simulink model "IBC_DCM_Test"  (R2019b)
settings: Solver=VariableStepAuto  StartTime=0.0  StopTime=0.03  RelTol=1e-3
InitFcn:
  | Load=2;
  | C=370e-6;
  | L1=1000e-6;
  | L2=1000e-6*(1+normrnd(0,0.05,[1,1]));
  | L3=1000e-6*(1+normrnd(0,0.05,[1,1]));
  | alp=1-0.5;
  | V = 12;
  | L = 1000e-6;
  | D = 0.5;
  | Vg= 12;
  | R = 2;
libraries: powerlib x23, simulink x12, dspsigops x5, powerlib_meascontrol x2
settings Model: SimulationMode=accelerator  Creator=29721  LastModifiedBy=29721

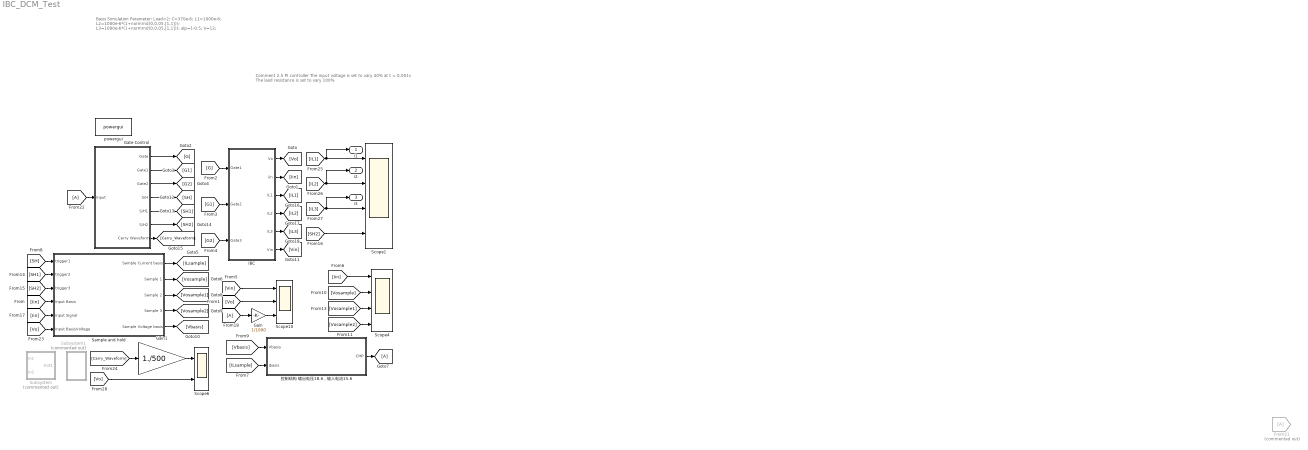
== system IBC_DCM_Test ==
  note: Comment 2.5
      | PI controller
      | The input voltage is set to vary 40% at t = 0.001s
      | The laod resistance is set to vary 100%
  note: Basis Simulation
      | Parameter:
      | Load=2;
      | C=370e-6;
      | L1=1000e-6;
      | L2=1000e-6*(1+normrnd(0,0.05,[1,1]));
      | L3=1000e-6*(1+normrnd(0,0.05,[1,1]));
      | alp=1-0.5;
      | V=12;
  From21 : From  Commented=on
  Gain : Gain  Gain=1/1000
  Gain1 : Gain  Gain=1./500
  Gate Control : Subsystem  mask{Fs=10e3}
      mask prompts: Fs "swicthing frequency"
  IBC : Subsystem  mask{L1=L1, L2=L1, L3=L1, C=C, R=R, Vin=Vg}
  "Sample and hold " : Subsystem
  Scope1 : Scope  NumInputPorts=4
  Scope10 : Scope  NumInputPorts=3
  Scope4 : Scope  NumInputPorts=4
  Scope6 : Scope  NumInputPorts=2
  Subsystem : Subsystem  Commented=on
  Subsystem1 : Subsystem  Commented=on
  powergui : powerlib/powergui  Priority=1  SimulationMode=Discrete  SampleTime=2.5e-8  frequency=60  Iterations=50  frequencyindice=0  Pbase=100e6  ErrMax=1e-4  UnitsV=kV  UnitsW=MW  buscounter=0  FunctionMessages=off  echomessages=off  EnableUseOfTLC=off  CurrentSourceSwitches=off  DisableSnubberDevices=off  DisableRonSwitches=off  DisableVfSwitches=off  DisplayEquations=off  AutomaticDiscreteSolvers=off  SolverType=Tustin/Backward Euler (TBE)  Interpol=off  ExternalGateDelay=off  methode=off  Ts=100  x0status=blocks  SPID=on  SwTol=0  HookPort=off  NonlinearTolerance=1e-4  nMaxIteration=100  ContinueOnMaxIteration=off  RestoreLinks=warning  ResistiveCurrentMeasurement=off  Frange=[0:2:500]  Ylog=off  Xlog=on  ShowGrid=off  save=off  variable=ZData  structure=0  ZoomFFT=off  StartTime=0.0  cycles=1  DisplayStyle=1  fundamental=60  FreqAxis=off  MaxFrequency=1000  frequencyindicesteady=1  RmsSteady=1  display=off
      settings: SourceProductName=Simscape Electrical
  控制结构 输出电压18.6，输入电流15.6 : Subsystem
  i1 : Outport
  i2 : Outport  Port=2
  i3 : Outport  Port=3
  wires:
  [Vosample1] -> Scope4/3
  [Vosample2] -> Scope4/4
  [Vin] -> Scope10/1
  [Vo] -> Scope10/2
  [Vosample] -> Scope4/2
  Gain1/1 -> Scope6/1
  [SH2] -> "Sample and hold "/3(trigger3)
  [Carry_Waveform] -> Gain1/1
  Gate Control/1(Gate) -> [G]
  Gate Control/2(Gate1) -> [G1]
  Gate Control/3(Gate2) -> [G2]
  [SH] -> "Sample and hold "/1(trigger1)
  [SH1] -> "Sample and hold "/2(trigger2)
  [Iin] -> "Sample and hold "/4(Input Basis)
  "Sample and hold "/1(Sample Current basis) -> [ILsample]
  "Sample and hold "/2(Sample 1) -> [Vosample]
  "Sample and hold "/3(Sample 2) -> [Vosample1]
  "Sample and hold "/4(Sample 3) -> [Vosample2]
  [Iin] -> Scope4/1
  [A] -> Gain/1
  "Sample and hold "/5(Sample Voltage basis) -> [Vbasis]
  [IL1] -> i1/1, Scope1/1
  [IL2] -> i2/1, Scope1/2
  [IL3] -> i3/1, Scope1/3
  [G] -> IBC/1(Gate1)
  [G1] -> IBC/2(Gate2)
  [G2] -> IBC/3(Gate3)
  IBC/1(Vo) -> [Vo]
  IBC/2(Iin) -> [Iin]
  [A] -> Gate Control/1(Input)
  Gate Control/4(S/H) -> [SH]
  Gate Control/5(S/H1) -> [SH1]
  Gate Control/6(S/H2) -> [SH2]
  [SH2] -> Scope1/4
  [Iin] -> "Sample and hold "/5(Input Signal)
  [Vo] -> "Sample and hold "/6(Input BasisVoltage)
  Gate Control/7(Carry Waveform) -> [Carry_Waveform]
  IBC/3(IL1) -> [IL1]
  IBC/4(IL2) -> [IL2]
  IBC/5(IL3) -> [IL3]
  [Vo] -> Scope6/2
  控制结构 输出电压18.6，输入电流15.6/1("CMP ") -> [A]
  [Vbasis] -> 控制结构 输出电压18.6，输入电流15.6/1(Vbasis)
  [ILsample] -> 控制结构 输出电压18.6，输入电流15.6/2(Ibasis)
  Gain/1 -> Scope10/3
  IBC/6(Vin) -> [Vin]

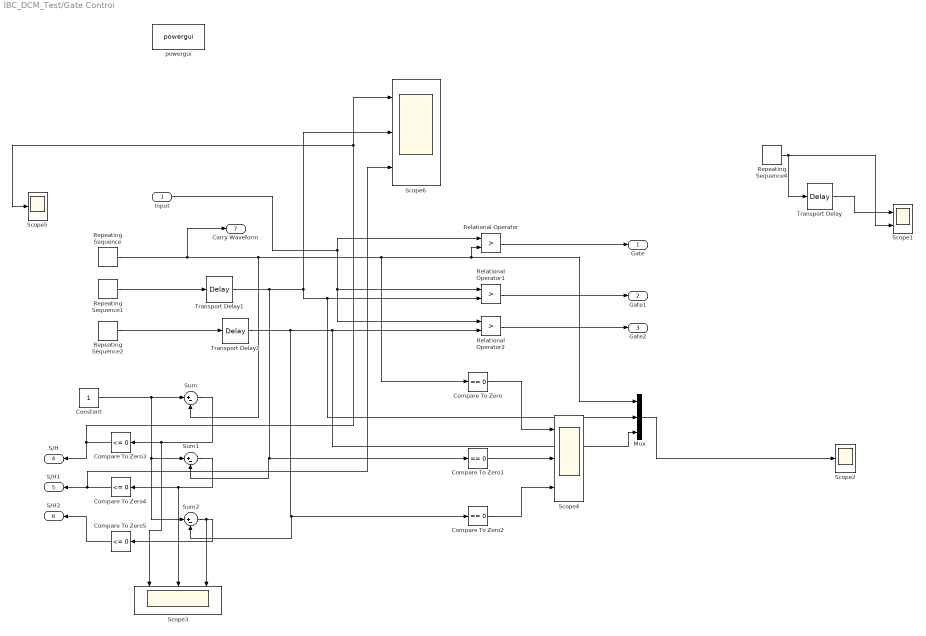
== system IBC_DCM_Test/Gate Control ==
  Input : Inport
  Compare To Zero : simulink/Logic and Bit Operations/Compare To Zero  relop===  OutDataTypeStr=boolean
  Compare To Zero1 : simulink/Logic and Bit Operations/Compare To Zero  relop===  OutDataTypeStr=boolean
  Compare To Zero2 : simulink/Logic and Bit Operations/Compare To Zero  relop===  OutDataTypeStr=boolean
  Compare To Zero3 : simulink/Logic and Bit Operations/Compare To Zero  relop=<=  OutDataTypeStr=boolean
  Compare To Zero4 : simulink/Logic and Bit Operations/Compare To Zero  relop=<=  OutDataTypeStr=boolean
  Compare To Zero5 : simulink/Logic and Bit Operations/Compare To Zero  relop=<=  OutDataTypeStr=boolean
  Constant : Constant
  Mux : Mux  Inputs=3
  Relational Operator : RelationalOperator  Operator=>  OutDataTypeStr=boolean  RndMeth=Simplest
  Relational Operator1 : RelationalOperator  Operator=>  OutDataTypeStr=boolean  RndMeth=Simplest
  Relational Operator2 : RelationalOperator  Operator=>  OutDataTypeStr=boolean  RndMeth=Simplest
  Repeating Sequence : simulink/Sources/Repeating Sequence  rep_seq_t=[0 1./Fs./2 1./Fs]  rep_seq_y=[0 1000 0]
  Repeating Sequence1 : simulink/Sources/Repeating Sequence  rep_seq_t=[1./Fs./3 5./Fs./6 4./Fs./3]  rep_seq_y=[0 1000 0]
  Repeating Sequence2 : simulink/Sources/Repeating Sequence  rep_seq_t=[2./Fs./3 7./Fs./6 5./Fs./3]  rep_seq_y=[0 1000 0]
  Repeating Sequence4 : simulink/Sources/Repeating Sequence  rep_seq_t=[0 1./100e3./2 1./100e3]  rep_seq_y=[0 1000 0]
  Scope1 : Scope  NumInputPorts=2
  Scope2 : Scope
  Scope3 : Scope  NumInputPorts=3
  Scope4 : Scope  NumInputPorts=3
  Scope5 : Scope
  Scope6 : Scope  NumInputPorts=3
  Sum : Sum  Inputs=|+-
  Sum1 : Sum  Inputs=|+-
  Sum2 : Sum  Inputs=|+-
  Transport Delay : TransportDelay  DelayTime=1./100e3./3
  Transport Delay1 : TransportDelay  DelayTime=1./Fs./3
  Transport Delay2 : TransportDelay  DelayTime=2./Fs./3
  powergui : powerlib/powergui  Priority=1  SimulationMode=Discrete  SampleTime=2.5e-8  frequency=60  Iterations=50  frequencyindice=60  Pbase=100e6  ErrMax=1e-4  UnitsV=kV  UnitsW=MW  buscounter=0  FunctionMessages=off  echomessages=off  EnableUseOfTLC=off  CurrentSourceSwitches=off  DisableSnubberDevices=off  DisableRonSwitches=off  DisableVfSwitches=off  DisplayEquations=off  AutomaticDiscreteSolvers=off  SolverType=Tustin/Backward Euler (TBE)  Interpol=off  ExternalGateDelay=off  methode=off  Ts=100  x0status=blocks  SPID=on  SwTol=0  HookPort=off  NonlinearTolerance=1e-4  nMaxIteration=100  ContinueOnMaxIteration=off  RestoreLinks=warning  ResistiveCurrentMeasurement=off  Frange=[0:2:500]  Ylog=off  Xlog=on  ShowGrid=off  save=off  variable=ZData  structure=0  ZoomFFT=off  StartTime=0.0  cycles=1  DisplayStyle=1  fundamental=60  FreqAxis=off  MaxFrequency=1000  frequencyindicesteady=1  RmsSteady=1  display=off
      settings: SourceProductName=Simscape Electrical
  Gate : Outport
  Gate1 : Outport  Port=2
  Gate2 : Outport  Port=3
  S/H : Outport  Port=4
  S/H1 : Outport  Port=5
  S/H2 : Outport  Port=6
  Carry Waveform : Outport  Port=7
  wires:
  Input/1 -> Relational Operator1/1, Relational Operator2/1, Relational Operator/1
  Compare To Zero/1 -> Scope4/1
  Relational Operator/1 -> Gate/1
  Repeating Sequence1/1 -> Transport Delay1/1
  Relational Operator1/1 -> Gate1/1
  Repeating Sequence2/1 -> Transport Delay2/1
  Repeating Sequence/1 -> Carry Waveform/1, Mux/1, Relational Operator/2, Compare To Zero/1, Sum/2
  Relational Operator2/1 -> Gate2/1
  Repeating Sequence4/1 -> Transport Delay/1, Scope1/2
  Transport Delay/1 -> Scope1/1
  Mux/1 -> Scope2/1
  Transport Delay1/1 -> Sum1/2, Compare To Zero1/1, Scope6/2, Mux/2, Relational Operator1/2
  Compare To Zero1/1 -> Scope4/2
  Compare To Zero2/1 -> Scope4/3
  Sum/1 -> Scope3/1, Compare To Zero3/1
  Sum1/1 -> Compare To Zero4/1, Scope3/2
  Transport Delay2/1 -> Sum2/2, Compare To Zero2/1, Mux/3, Relational Operator2/2
  Sum2/1 -> Scope3/3, Compare To Zero5/1
  Constant/1 -> Sum2/1, Sum1/1, Sum/1
  Compare To Zero3/1 -> Scope6/1, Scope5/1, S/H/1
  Compare To Zero4/1 -> Scope6/3, S/H1/1
  Compare To Zero5/1 -> S/H2/1

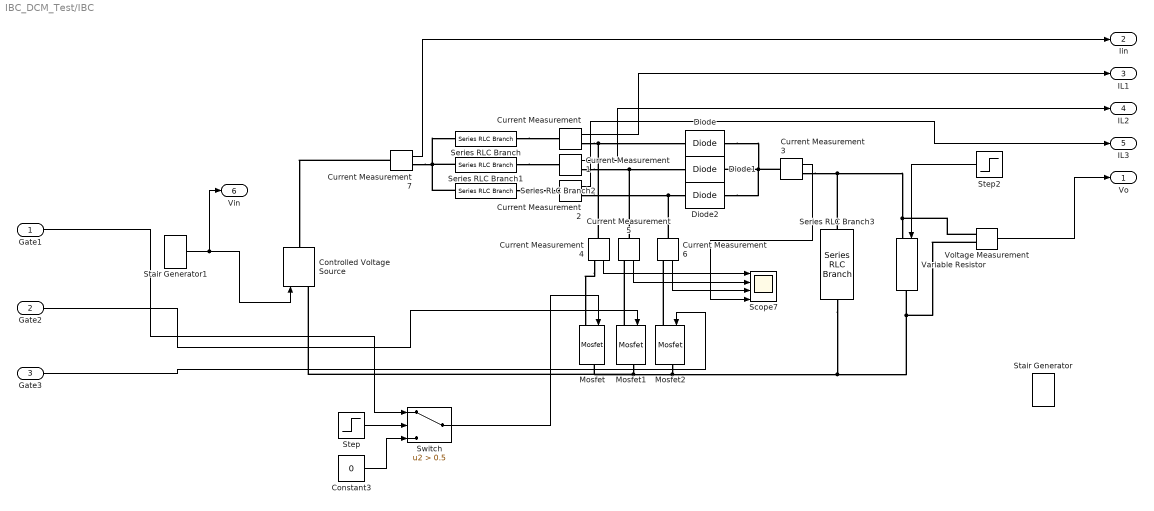
== system IBC_DCM_Test/IBC ==
  Gate1 : Inport
  Gate2 : Inport  Port=2
  Gate3 : Inport  Port=3
  Constant3 : Constant  Value=0
  Controlled Voltage Source : powerlib/Electrical Sources/Controlled Voltage Source  Initialize=on  Source_Type=AC  Amplitude=0  Phase=0  Frequency=0  Measurements=None
      settings: SourceProductName=Simscape Electrical
  Current Measurement{,1..7} (8 alike) : powerlib/Measurements/Current Measurement  PhasorSimulation=off  OutputType=Complex  PSBequivalent=0
      settings: SourceProductName=Simscape Electrical
  Diode : powerlib/Power Electronics/Diode  Ron=0.001  Lon=0  Vf=0  IC=0  UseSnubber=0  Rs=inf  Cs=250e-9  Measurements=off
      settings: SourceProductName=Simscape Electrical
  Diode1 : powerlib/Power Electronics/Diode  Ron=0.001  Lon=0  Vf=0  IC=0  UseSnubber=0  Rs=inf  Cs=250e-9  Measurements=off
      settings: SourceProductName=Simscape Electrical
  Diode2 : powerlib/Power Electronics/Diode  Ron=0.001  Lon=0  Vf=0  IC=0  UseSnubber=0  Rs=inf  Cs=250e-9  Measurements=off
      settings: SourceProductName=Simscape Electrical
  Mosfet : powerlib/Power Electronics/Mosfet  Ron=0.01  Lon=0  Rd=0.01  Vfd=0  IC=0  Rs=1e5  Cs=inf  Measurements=off
      settings: SourceProductName=Simscape Electrical
  Mosfet1 : powerlib/Power Electronics/Mosfet  Ron=0.01  Lon=0  Rd=0.01  Vfd=0  IC=0  Rs=1e5  Cs=inf  Measurements=off
      settings: SourceProductName=Simscape Electrical
  Mosfet2 : powerlib/Power Electronics/Mosfet  Ron=0.01  Lon=0  Rd=0.01  Vfd=0  IC=0  Rs=1e5  Cs=inf  Measurements=off
      settings: SourceProductName=Simscape Electrical
  Scope7 : Scope  NumInputPorts=4
  Series RLC Branch : powerlib/Elements/Series RLC Branch  LConnTagsString=__new0  RConnTagsString=__new0  BranchType=L  Resistance=1  Inductance=L1  SetiL0=off  InitialCurrent=0  Capacitance=1e-6  Setx0=off  InitialVoltage=0  Measurements=None
      settings: SourceProductName=Simscape Electrical
  Series RLC Branch1 : powerlib/Elements/Series RLC Branch  LConnTagsString=__new0  RConnTagsString=__new0  BranchType=L  Resistance=1  Inductance=L2  SetiL0=off  InitialCurrent=0  Capacitance=1e-6  Setx0=off  InitialVoltage=0  Measurements=None
      settings: SourceProductName=Simscape Electrical
  Series RLC Branch2 : powerlib/Elements/Series RLC Branch  LConnTagsString=__new0  RConnTagsString=__new0  BranchType=L  Resistance=1  Inductance=L3  SetiL0=off  InitialCurrent=0  Capacitance=1e-6  Setx0=off  InitialVoltage=0  Measurements=None
      settings: SourceProductName=Simscape Electrical
  Series RLC Branch3 : powerlib/Elements/Series RLC Branch  LConnTagsString=__new0  RConnTagsString=__new0  BranchType=RC  Resistance=0  Inductance=1e-3  SetiL0=off  InitialCurrent=0  Capacitance=C  Setx0=off  InitialVoltage=0  Measurements=None
      settings: SourceProductName=Simscape Electrical
  Stair Generator : powerlib_meascontrol/Pulse & Signal Generators/Stair Generator  t=[0,0.01,0.02]  e=[2,4,8]  Ts=0
      settings: SourceProductName=Simscape Electrical
  Stair Generator1 : powerlib_meascontrol/Pulse & Signal Generators/Stair Generator  t=[0,0.01,0.02]  e=[10,10,10]  Ts=0
      settings: SourceProductName=Simscape Electrical
  Step : Step  Time=0.025  Before=1  After=0  SampleTime=0
  Step2 : Step  Time=0.01  Before=4  After=6  SampleTime=0
  Switch : Switch  Criteria=u2 > Threshold  Threshold=0.5
  Variable Resistor : powerlib/Elements/Variable Resistor  Rabsmin=1e-3
      settings: SourceProductName=Simscape Electrical  SourceProductBaseCode=PS
  Voltage Measurement : powerlib/Measurements/Voltage Measurement  PhasorSimulation=off  OutputType=Complex  PSBequivalent=0
      settings: SourceProductName=Simscape Electrical
  Vo : Outport
  Iin : Outport  Port=2
  IL1 : Outport  Port=3
  IL2 : Outport  Port=4
  IL3 : Outport  Port=5
  Vin : Outport  Port=6
  wires:
  Step2/1 -> Variable Resistor/1
  Current Measurement6/1 -> Scope7/3
  Current Measurement5/1 -> Scope7/2
  Current Measurement1/1 -> IL2/1
  Current Measurement4/1 -> Scope7/1
  Current Measurement2/1 -> IL3/1
  Step/1 -> Switch/2
  Switch/1 -> Mosfet/1
  Current Measurement3/1 -> Scope7/4
  Stair Generator1/1 -> Vin/1, Controlled Voltage Source/1
  Gate3/1 -> Mosfet2/1
  Voltage Measurement/1 -> Vo/1
  Current Measurement/1 -> IL1/1
  Constant3/1 -> Switch/3
  Current Measurement7/1 -> Iin/1
  Gate1/1 -> Switch/1
  Gate2/1 -> Mosfet1/1
  connections:
  Series RLC Branch2/RConn1 -- Current Measurement2/LConn1
  Mosfet2/LConn1 -- Current Measurement6/RConn1
  Current Measurement7/LConn1 -- Controlled Voltage Source/RConn1
  Series RLC Branch/RConn1 -- Current Measurement/LConn1
  Series RLC Branch1/RConn1 -- Current Measurement1/LConn1
  Controlled Voltage Source/LConn1 -- Mosfet/RConn1 -- Mosfet1/RConn1 -- Mosfet2/RConn1 -- Voltage Measurement/LConn2 -- Variable Resistor/RConn1 -- Series RLC Branch3/RConn1
  Mosfet1/LConn1 -- Current Measurement5/RConn1
  Current Measurement2/RConn1 -- Current Measurement6/LConn1 -- Diode2/LConn1
  Current Measurement3/RConn1 -- Series RLC Branch3/LConn1 -- Voltage Measurement/LConn1 -- Variable Resistor/LConn1
  Current Measurement4/RConn1 -- Mosfet/LConn1
  Current Measurement7/RConn1 -- Series RLC Branch2/LConn1 -- Series RLC Branch1/LConn1 -- Series RLC Branch/LConn1
  Current Measurement1/RConn1 -- Diode1/LConn1 -- Current Measurement5/LConn1
  Current Measurement3/LConn1 -- Diode2/RConn1 -- Diode/RConn1 -- Diode1/RConn1
  Current Measurement/RConn1 -- Diode/LConn1 -- Current Measurement4/LConn1

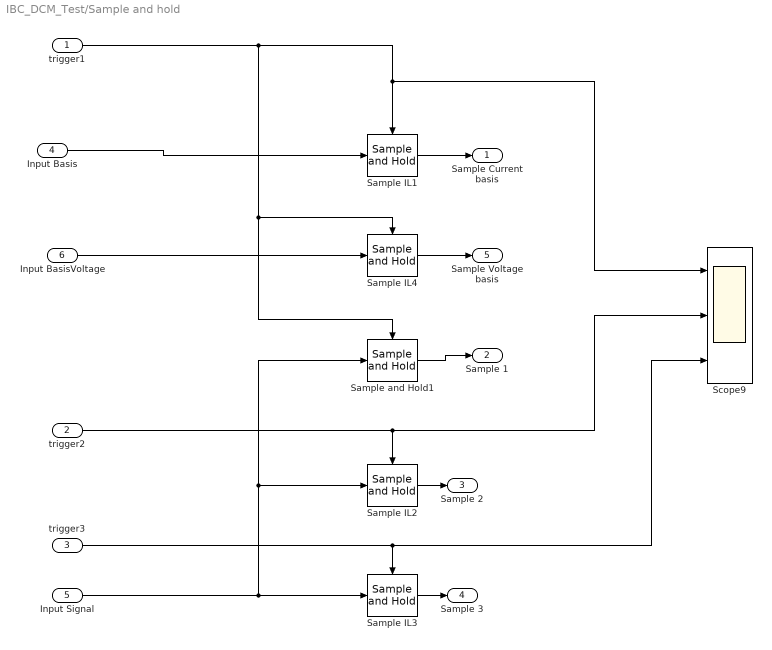
== system IBC_DCM_Test/Sample and hold  ==
  trigger1 : Inport
  trigger2 : Inport  Port=2
  trigger3 : Inport  Port=3
  Input Basis : Inport  Port=4
  Input Signal : Inport  Port=5
  Input BasisVoltage : Inport  Port=6
  Sample IL{1..4} (4 alike) : dspsigops/Sample and Hold  trig=Rising edge  initCond=0  latchinput=off
  Sample and Hold1 : dspsigops/Sample and Hold  trig=Rising edge  initCond=0  latchinput=off
  Scope9 : Scope  NumInputPorts=3
  Sample Current basis : Outport
  Sample 1 : Outport  Port=2
  Sample 2 : Outport  Port=3
  Sample 3 : Outport  Port=4
  Sample Voltage basis : Outport  Port=5
  wires:
  trigger3/1 -> Sample IL3/Trigger, Scope9/3
  Input Signal/1 -> Sample and Hold1/1, Sample IL2/1, Sample IL3/1
  Sample IL3/1 -> Sample 3/1
  trigger1/1 -> Scope9/1, Sample IL1/Trigger, Sample IL4/Trigger, Sample and Hold1/Trigger
  trigger2/1 -> Sample IL2/Trigger, Scope9/2
  Sample IL2/1 -> Sample 2/1
  Input Basis/1 -> Sample IL1/1
  Sample IL1/1 -> Sample Current basis/1
  Sample and Hold1/1 -> Sample 1/1
  Input BasisVoltage/1 -> Sample IL4/1
  Sample IL4/1 -> Sample Voltage basis/1

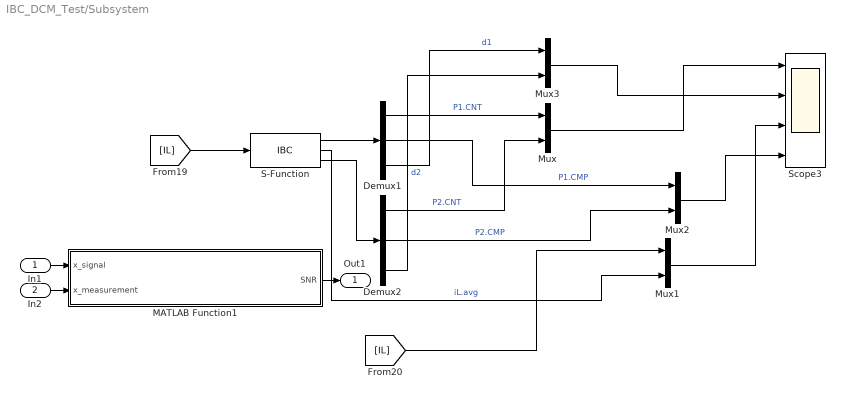
== system IBC_DCM_Test/Subsystem ==
  In1 : Inport
  In2 : Inport  Port=2
  Demux1 : Demux  Outputs=3
  Demux2 : Demux  Outputs=3
  MATLAB Function1 : MATLAB Function  TreatAsAtomicUnit=on
  Mux{,1..3} (4 alike) : Mux  Inputs=2
  S-Function : S-Function  FunctionName=IBC  SFunctionDeploymentMode=off  EnableBusSupport=off
  Scope3 : Scope  NumInputPorts=4
  Out1 : Outport
  wires:
  Demux1/2 -> Mux2/1  "P1.CMP"
  In2/1 -> MATLAB Function1/2(x_measurement)
  S-Function/3 -> Demux2/1
  Mux2/1 -> Scope3/4
  [IL] -> Mux1/1
  Demux1/1 -> Mux/1  "P1.CNT"
  S-Function/2 -> Mux1/2  "iL.avg"
  Demux2/3 -> Mux3/2  "d2"
  Mux1/1 -> Scope3/3
  S-Function/1 -> Demux1/1
  Mux/1 -> Scope3/1
  In1/1 -> MATLAB Function1/1(x_signal)
  Demux2/1 -> Mux/2  "P2.CNT"
  Demux1/3 -> Mux3/1  "d1"
  [IL] -> S-Function/1
  Demux2/2 -> Mux2/2  "P2.CMP"
  Mux3/1 -> Scope3/2
  MATLAB Function1/1(SNR) -> Out1/1

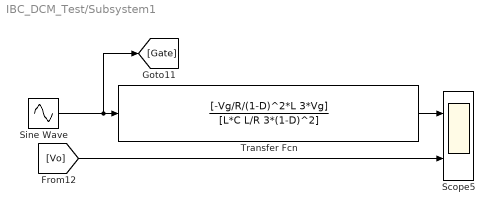
== system IBC_DCM_Test/Subsystem1 ==
  Scope5 : Scope  NumInputPorts=2
  Sine Wave : Sin  Amplitude=0.05  Bias=0.5  Frequency=2*pi*8e3  SampleTime=0
  Transfer Fcn : TransferFcn  Numerator=[-Vg/R/(1-D)^2*L 3*Vg]  Denominator=[L*C L/R 3*(1-D)^2]
  wires:
  [Vo] -> Scope5/2
  Transfer Fcn/1 -> Scope5/1
  Sine Wave/1 -> Transfer Fcn/1, [Gate]

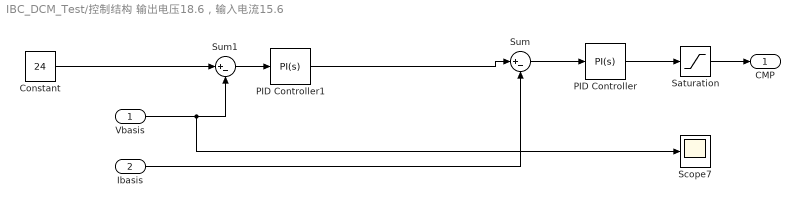
== system IBC_DCM_Test/控制结构 输出电压18.6，输入电流15.6 ==
  Vbasis : Inport
  Ibasis : Inport  Port=2
  Constant : Constant  Value=24
  PID Controller : simulink/Continuous/PID Controller  Controller=PI  Form=Parallel  TimeDomain=Continuous-time  SampleTime=-1  IntegratorMethod=Forward Euler  FilterMethod=Forward Euler  ControllerParametersSource=internal  P=77.738292364102001535116841188175  I=38432.721244442002763594847678325  D=0  UseFilter=on  N=100  TunerSelectOption=Transfer Function Based (PID Tuner App)  InitialConditionSource=internal  InitialConditionForIntegrator=0  InitialConditionForFilter=0  DifferentiatorICPrevScaledInput=0  ExternalReset=none  TrackingMode=off  Kt=1  LimitOutput=off  UpperSaturationLimit=inf  LowerSaturationLimit=-inf  LinearizeAsGain=on  AntiWindupMode=none  Kb=1  POutMin=[]  POutMax=[]  IOutMin=[]  IOutMax=[]  DOutMin=[]  DOutMax=[]  NOutMin=[]  NOutMax=[]  SumOutMin=[]  SumOutMax=[]  SaturationOutMin=[]  SaturationOutMax=[]  PParamMin=[]  PParamMax=[]  IParamMin=[]  IParamMax=[]  DParamMin=[]  DParamMax=[]  NParamMin=[]  NParamMax=[]  KbParamMin=[]  KbParamMax=[]  KtParamMin=[]  KtParamMax=[]  KbOutMin=[]  KbOutMax=[]  KtOutMin=[]  KtOutMax=[]  IntegratorOutMin=[]  IntegratorOutMax=[]  FilterOutMin=[]  FilterOutMax=[]  SumI1OutMin=[]  SumI1OutMax=[]  SumI2OutMin=[]  SumI2OutMax=[]  SumI3OutMin=[]  SumI3OutMax=[]  SumI4OutMin=[]  SumI4OutMax=[]  SumDOutMin=[]  SumDOutMax=[]  DifferentiatorOutMin=[]  DifferentiatorOutMax=[]  FilterDiffOutCoefMin=[]  FilterDiffOutCoefMax=[]  ReciprocalOutMin=[]  ReciprocalOutMax=[]  SumDenOutMin=[]  SumDenOutMax=[]  SumNumOutMin=[]  SumNumOutMax=[]  DivideOutMin=[]  DivideOutMax=[]  IntegratorContinuousStateAttributes=''  IntegratorStateMustResolveToSignalObject=off  IntegratorRTWStateStorageClass=Auto  FilterContinuousStateAttributes=''  FilterStateMustResolveToSignalObject=off  FilterRTWStateStorageClass=Auto  ParallelPVariant=InternalParameters  IdealPVariant=Disabled  IVariant=InternalParameters  DVariant=Disabled  IntegratorVariant=Continuous  SatVariant=Disabled  AWVariant=Passthrough  PCopyVariant=Disabled  TRVariant=Disabled  FdbkBlocksVariant=Forward  IdealPFdbkVariant=Disabled  SatFdbkVariant=Disabled  DerivativeFilterVariant=Disabled  NVariant=Disabled  NCopyVariant=Disabled_SignalSpec  FilterICVariant=Disabled  IntegratorICVariant=InternalICs  ExternalResetVariant=Disabled  TRSumVariant=Passthrough  SumFdbkVariant=Disabled  SumVariant=Sum_PI
  PID Controller1 : simulink/Continuous/PID Controller  Controller=PI  Form=Parallel  TimeDomain=Continuous-time  SampleTime=-1  IntegratorMethod=Forward Euler  FilterMethod=Forward Euler  ControllerParametersSource=internal  P=0.62718109879312408739947745769878  I=971.09450057614076065122020625338  D=0  UseFilter=on  N=100  TunerSelectOption=Transfer Function Based (PID Tuner App)  InitialConditionSource=internal  InitialConditionForIntegrator=0  InitialConditionForFilter=0  DifferentiatorICPrevScaledInput=0  ExternalReset=none  TrackingMode=off  Kt=1  LimitOutput=off  UpperSaturationLimit=inf  LowerSaturationLimit=-inf  LinearizeAsGain=on  AntiWindupMode=none  Kb=1  POutMin=[]  POutMax=[]  IOutMin=[]  IOutMax=[]  DOutMin=[]  DOutMax=[]  NOutMin=[]  NOutMax=[]  SumOutMin=[]  SumOutMax=[]  SaturationOutMin=[]  SaturationOutMax=[]  PParamMin=[]  PParamMax=[]  IParamMin=[]  IParamMax=[]  DParamMin=[]  DParamMax=[]  NParamMin=[]  NParamMax=[]  KbParamMin=[]  KbParamMax=[]  KtParamMin=[]  KtParamMax=[]  KbOutMin=[]  KbOutMax=[]  KtOutMin=[]  KtOutMax=[]  IntegratorOutMin=[]  IntegratorOutMax=[]  FilterOutMin=[]  FilterOutMax=[]  SumI1OutMin=[]  SumI1OutMax=[]  SumI2OutMin=[]  SumI2OutMax=[]  SumI3OutMin=[]  SumI3OutMax=[]  SumI4OutMin=[]  SumI4OutMax=[]  SumDOutMin=[]  SumDOutMax=[]  DifferentiatorOutMin=[]  DifferentiatorOutMax=[]  FilterDiffOutCoefMin=[]  FilterDiffOutCoefMax=[]  ReciprocalOutMin=[]  ReciprocalOutMax=[]  SumDenOutMin=[]  SumDenOutMax=[]  SumNumOutMin=[]  SumNumOutMax=[]  DivideOutMin=[]  DivideOutMax=[]  IntegratorContinuousStateAttributes=''  IntegratorStateMustResolveToSignalObject=off  IntegratorRTWStateStorageClass=Auto  FilterContinuousStateAttributes=''  FilterStateMustResolveToSignalObject=off  FilterRTWStateStorageClass=Auto  ParallelPVariant=InternalParameters  IdealPVariant=Disabled  IVariant=InternalParameters  DVariant=Disabled  IntegratorVariant=Continuous  SatVariant=Disabled  AWVariant=Passthrough  PCopyVariant=Disabled  TRVariant=Disabled  FdbkBlocksVariant=Forward  IdealPFdbkVariant=Disabled  SatFdbkVariant=Disabled  DerivativeFilterVariant=Disabled  NVariant=Disabled  NCopyVariant=Disabled_SignalSpec  FilterICVariant=Disabled  IntegratorICVariant=InternalICs  ExternalResetVariant=Disabled  TRSumVariant=Passthrough  SumFdbkVariant=Disabled  SumVariant=Sum_PI
  Saturation : Saturate  UpperLimit=1000  LowerLimit=0
  Scope7 : Scope
  Sum : Sum  Inputs=|+-
  Sum1 : Sum  Inputs=|+-
  "CMP " : Outport
  wires:
  Ibasis/1 -> Sum/2
  Sum1/1 -> PID Controller1/1
  Sum/1 -> PID Controller/1
  Vbasis/1 -> Scope7/1, Sum1/2
  Saturation/1 -> "CMP "/1
  PID Controller/1 -> Saturation/1
  PID Controller1/1 -> Sum/1
  Constant/1 -> Sum1/1

== matlab function IBC_DCM_Test/Subsystem/MATLAB Function1 ==
  data: x_signal input; SNR output; x_measurement input
function SNR = SNR_calculte(x_signal,x_measurement)
%================== Calculate the SNR ===================%
x_noise = x_measurement-x_signal;
% Calculate the power of the signal and noise
Ps = sum(x_signal.^2)./length(x_signal);
Pn = sum(x_noise.^2)./length(x_noise);
% Calculate the SNR
SNR = 10*log10(Ps/Pn);
